simulink model "MotorSpeedAnalysisLAST"  (R2016a)
settings: Solver=ode4  SolverMode=SingleTasking  StartTime=0.0  StopTime=150  FixedStep=Ts  RelTol=1e-3
undefined symbols (not defined in the file or in its folder): Ts
libraries: arduino_io_lib x3
settings Model: ExtModeTrigDuration=2  Creator=gcampa  LastModifiedBy=syf
settings DataIOCC: LimitDataPoints=on  SaveFormat=Array  SignalLoggingSaveFormat=ModelDataLogs
settings OptimizationCC: OptimizeModelRefInitCode=on  LifeSpan=1  MaxStackSize=64
settings DebuggingCC: UnderspecifiedInitializationDetection=Classic  MergeDetectMultiDrivingBlocksExec=none  MultiTaskDSMMsg=warning  MultiTaskCondExecSysMsg=none
settings HardwareCC: ProdBitPerInt=16  ProdBitPerPointer=16  ProdLargestAtomicFloat=None  ProdWordSize=8  ProdHWDeviceType=Atmel->AVR
settings ModelReferenceCC: PropagateSignalLabelsOutOfModel=off
settings RTWCC: SystemTargetFile=ert.tlc  HardwareBoard=Arduino Uno  TemplateMakefile=ert_default_tmf  GenerateReport=on  RTWVerbose=off  Toolchain=Arduino AVR v1.6.1  BuildConfiguration=Faster Runs  IncludeHyperlinkInReport=on  LaunchReport=on  GenerateTraceInfo=on  GenerateTraceReport=on  GenerateTraceReportSl=on  GenerateTraceReportSf=on  GenerateTraceReportEml=on
settings CodeAppCC: ForceParamTrailComments=on  IgnoreCustomStorageClasses=off  OperatorAnnotations=on  SimulinkDataObjDesc=on  SFDataObjDesc=on  MATLABFcnDesc=on  InsertBlockDesc=on  MATLABSourceComments=on
settings ERTTargetCC: SupportContinuousTime=on  SupportVariableSizeSignals=on
settings ConfigComp: CovModelRefEnable=Off

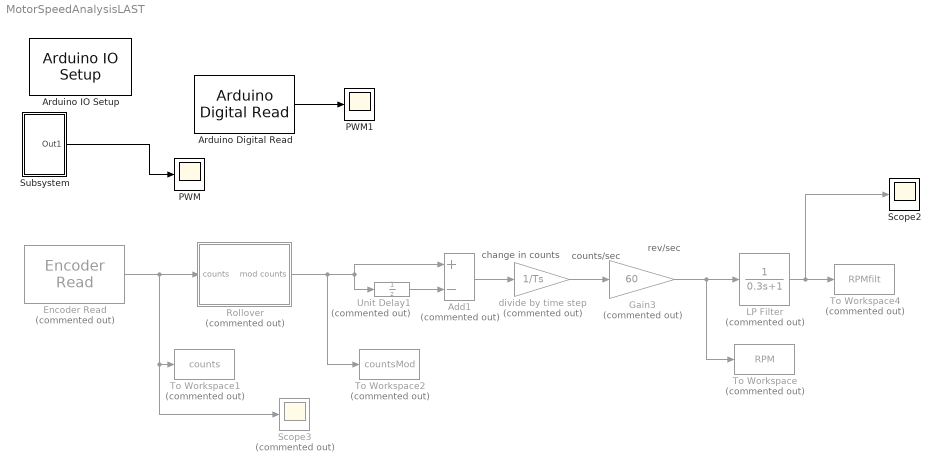
== system MotorSpeedAnalysisLAST ==
  note: change
      | in counts
  note: rev/sec
  note: counts/sec
  Add1 : Sum  Commented=on  Inputs=+-
  Arduino Digital Read : arduino_io_lib/Arduino Digital Read  arduinoVar=Temporary arduino variable: Arduino1  arduinoPin=6  T=0.2
  Arduino IO Setup : arduino_io_lib/Arduino IO Setup  Priority=3  arduinoVar=Temporary arduino variable: Arduino1  workspaceVarName=a  comPort=COM5
  Encoder Read : arduino_io_lib/Encoder Read  Commented=on  arduinoVar=Temporary arduino variable: Arduino1  encNum=2  pinA=3  pinB=2  DbDl=0  T=Ts
  Gain3 : Gain  Commented=on  Gain=60
  LP Filter : TransferFcn  Commented=on  Denominator=[0.3 1]
  PWM : Scope
  PWM1 : Scope
  Rollover : Subsystem  Commented=on
  Scope2 : Scope
  Scope3 : Scope  Commented=on
  Subsystem : Subsystem
  To Workspace : ToWorkspace  Commented=on  VariableName=RPM  SaveFormat=Timeseries  SampleTime=-1
  To Workspace1 : ToWorkspace  Commented=on  VariableName=counts  SaveFormat=Timeseries  SampleTime=-1
  To Workspace2 : ToWorkspace  Commented=on  VariableName=countsMod  SaveFormat=Timeseries  SampleTime=-1
  To Workspace4 : ToWorkspace  Commented=on  VariableName=RPMfilt  SaveFormat=Timeseries  SampleTime=-1
  Unit Delay1 : UnitDelay  Commented=on  SampleTime=-1
  divide by time step : Gain  Commented=on  Gain=1/Ts
  wires:
  Unit Delay1/1 -> Add1/2
  divide by time step/1 -> Gain3/1
  Add1/1 -> divide by time step/1
  Rollover/1(" mod counts") -> To Workspace2/1, Add1/1, Unit Delay1/1
  Encoder Read/1 -> Scope3/1, To Workspace1/1, Rollover/1(counts)
  Subsystem/1(Out1) -> PWM/1
  Gain3/1 -> To Workspace/1, LP Filter/1
  LP Filter/1 -> Scope2/1, To Workspace4/1
  Arduino Digital Read/1 -> PWM1/1

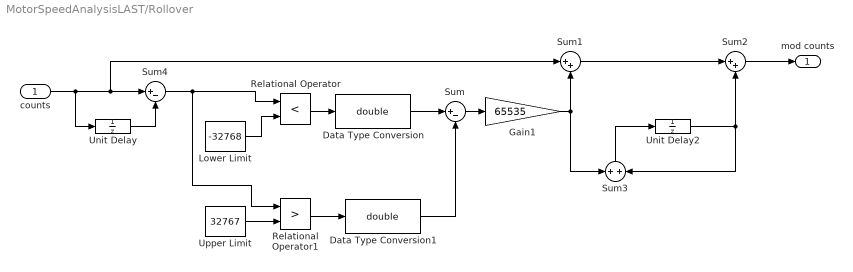
== system MotorSpeedAnalysisLAST/Rollover ==
  counts : Inport
  " Lower Limit" : Constant  Value=-32768
  " Upper Limit" : Constant  Value=32767
  Data Type Conversion : DataTypeConversion  OutDataTypeStr=double  RndMeth=Zero
  Data Type Conversion1 : DataTypeConversion  OutDataTypeStr=double  RndMeth=Zero
  Gain1 : Gain  Gain=65535
  Relational Operator : RelationalOperator  Operator=<  OutDataTypeStr=boolean
  Relational Operator1 : RelationalOperator  Operator=>  OutDataTypeStr=boolean
  Sum : Sum  Inputs=|+-
  Sum1 : Sum  Inputs=|++
  Sum2 : Sum  Inputs=|++
  Sum3 : Sum
  Sum4 : Sum  Inputs=|+-
  Unit Delay : UnitDelay  SampleTime=-1
  Unit Delay2 : UnitDelay  SampleTime=-1
  " mod counts" : Outport
  wires:
  counts/1 -> Unit Delay/1, Sum1/1, Sum4/1
  Sum2/1 -> " mod counts"/1
  Unit Delay/1 -> Sum4/2
  Data Type Conversion/1 -> Sum/1
  Sum3/1 -> Unit Delay2/1
  Data Type Conversion1/1 -> Sum/2
  Sum/1 -> Gain1/1
  Gain1/1 -> Sum1/2, Sum3/1
  Relational Operator1/1 -> Data Type Conversion1/1
  Sum1/1 -> Sum2/1
  Relational Operator/1 -> Data Type Conversion/1
  " Upper Limit"/1 -> Relational Operator1/2
  Unit Delay2/1 -> Sum3/2, Sum2/2
  " Lower Limit"/1 -> Relational Operator/2
  Sum4/1 -> Relational Operator/1, Relational Operator1/1

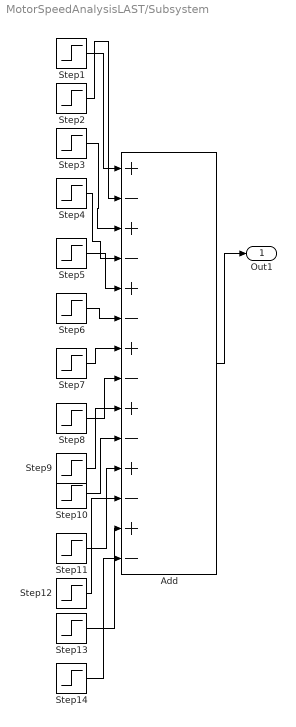
== system MotorSpeedAnalysisLAST/Subsystem ==
  Add : Sum  Inputs=+-+-+-+-+-+-+-
  Step1 : Step  Time=3  SampleTime=0
  Step10 : Step  Time=77  SampleTime=0
  Step11 : Step  Time=86  SampleTime=0
  Step12 : Step  Time=100  SampleTime=0
  Step13 : Step  Time=120  SampleTime=0
  Step14 : Step  Time=135  SampleTime=0
  Step2 : Step  Time=13  SampleTime=0
  Step3 : Step  Time=18  SampleTime=0
  Step4 : Step  Time=27  SampleTime=0
  Step5 : Step  Time=40  SampleTime=0
  Step6 : Step  Time=44  SampleTime=0
  Step7 : Step  Time=51  SampleTime=0
  Step8 : Step  Time=67  SampleTime=0
  Step9 : Step  Time=74  SampleTime=0
  Out1 : Outport
  wires:
  Step4/1 -> Add/4
  Step7/1 -> Add/7
  Step3/1 -> Add/3
  Step8/1 -> Add/8
  Step5/1 -> Add/5
  Step1/1 -> Add/1
  Add/1 -> Out1/1
  Step6/1 -> Add/6
  Step2/1 -> Add/2
  Step9/1 -> Add/9
  Step14/1 -> Add/14
  Step11/1 -> Add/11
  Step13/1 -> Add/13
  Step10/1 -> Add/10
  Step12/1 -> Add/12
